simulink model "Poten"  (R2024b)
settings: Solver=FixedStepAuto  StartTime=0.0  StopTime=inf  RelTol=1e-3  EnableMultiTasking=on
libraries: stm32f4xxblockslib x2, simulink x1
settings Model: STM32="{\"AnalogInput\":[{\"ID\":\"untitled:1\"},{\"ID\":\"Poten:1\"}],\"DigitalPortRead\":[{\"ID\":\"untitled:21\"},{\"ID\":\"Poten:21\"}]}"  Creator=rew1m  LastModifiedBy=janej
settings OptimizationCC: DefaultParameterBehavior=Inlined  EnhancedBackFolding=on  PassReuseOutputArgsAs=Individual arguments  ZeroExternalMemoryAtStartup=off  ZeroInternalMemoryAtStartup=off  MaxStackSize=512  OptimizeBlockOrder=speed  DifferentSizesBufferReuse=on  OptimizationCustomize=off  EfficientTunableParamExpr=on
settings DebuggingCC: ParameterTunabilityLossMsg=error
settings HardwareCC: ProdBitPerPointer=32  ProdBitPerSizeT=32  ProdBitPerPtrDiffT=32  ProdLargestAtomicInteger=Long  ProdLargestAtomicFloat=Double  ProdWordSize=32  ProdLongLongMode=on  ProdHWDeviceType=ARM Compatible->ARM Cortex-M
settings SFSimCC: MATLABDynamicMemAlloc=off
settings RTWCC: Description=Embedded Coder  SystemTargetFile=ert.tlc  HardwareBoard=STM32G4xx Based  TemplateMakefile=ert_default_tmf  Toolchain=GNU Tools for ARM Embedded Processors
settings CodeAppCC: ForceParamTrailComments=on  IgnoreCustomStorageClasses=off  OperatorAnnotations=on  SimulinkDataObjDesc=on  SFDataObjDesc=on  InsertBlockDesc=on
settings ERTTargetCC: TargetLangStandard=C99 (ISO)  CodeReplacementLibrary=ARM Cortex-M  ExtModeTransport=3  ExtModeStaticAlloc=on  ExtModeStaticAllocSize=2048  ExtModeMexFile=ext_xcp  ExtModeIntrfLevel=Level2 - Open

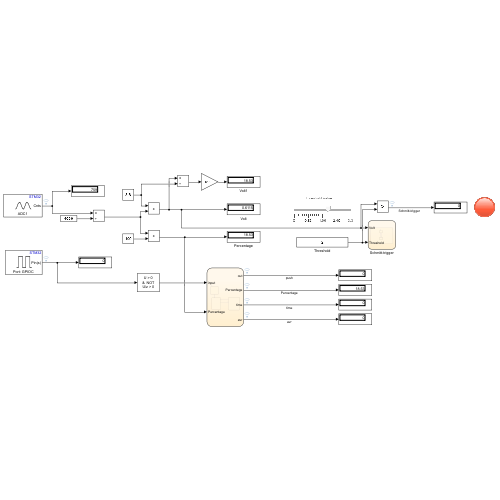
[thumbnail: Simulink's stored preview of the top-level diagram]
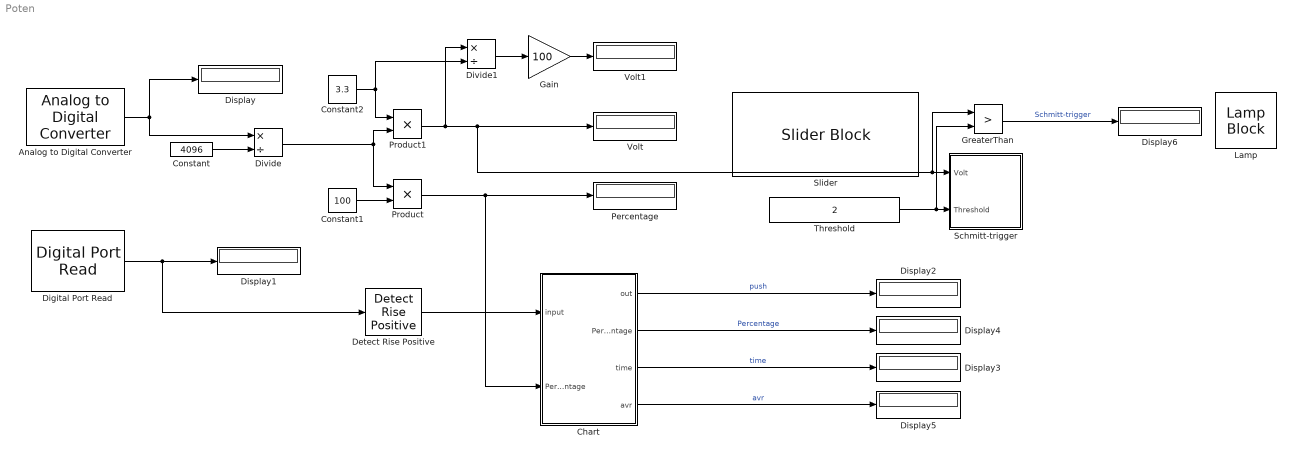
== system Poten ==
  Analog to Digital Converter : stm32f4xxblockslib/Analog to Digital Converter  ADCModule=ADC1  ConversionGroup=Regular  TriggerMode=Trigger and read  NumberOfConversions=1  EnableBufferConv=off  BufferLength=1  OutputStatus=off  SampleTime=-1  EnableSimPort=off  hoistedMaskSrc=ECSoC/ECSimCodegen/Analog to Digital Converter
  Chart : Stateflow chart  TreatAsAtomicUnit=on
  Constant : Constant  Value=4096
  Constant1 : Constant  Value=100
  Constant2 : Constant  Value=3.3
  Detect Rise Positive : simulink/Logic and Bit Operations/Detect Rise Positive  vinit=0  OutDataTypeStr=boolean
  Digital Port Read : stm32f4xxblockslib/Digital Port Read  PortName=GPIOC  PinNumber=[13]  ReadOperation=on  IOAsArray=on  SampleTime=-1  EnableSimPort=off  hoistedMaskSrc=ECSoC/ECSimCodegen/Digital Port Read
  Display{,1..6} (7 alike) : Display
  Divide : Product  Inputs=*/
  Divide1 : Product  Inputs=*/
  Gain : Gain  Gain=100
  GreaterThan : RelationalOperator  Operator=>  OutDataTypeStr=boolean  RndMeth=Simplest  InputSameDT=off
  Lamp : LampBlock  LabelPosition=Hide
  Percentage : Display
  Product : Product
  Product1 : Product
  Schmitt-trigger : Stateflow chart  TreatAsAtomicUnit=on
  Slider : SliderBlock  ScaleMax=3.3
  Threshold : Constant  Value=2
  Volt : Display
  Volt1 : Display
  wires:
  Analog to Digital Converter/1 -> Display/1, Divide/1
  Constant/1 -> Divide/2
  Divide/1 -> Product/1, Product1/2
  Constant1/1 -> Product/2
  Product/1 -> Chart/2("Percentage "), Percentage/1
  Constant2/1 -> Product1/1, Divide1/2
  Product1/1 -> GreaterThan/1, Schmitt-trigger/1(Volt), Volt/1, Divide1/1
  Divide1/1 -> Gain/1
  Gain/1 -> Volt1/1
  Digital Port Read/1 -> Detect Rise Positive/1, Display1/1
  Detect Rise Positive/1 -> Chart/1(input)
  Chart/1(out) -> Display2/1  "push"
  Chart/3(time) -> Display3/1  "time"
  GreaterThan/1 -> Display6/1  "Schmitt-trigger"
  Threshold/1 -> GreaterThan/2, Schmitt-trigger/2(Threshold)
  Chart/2(Percentage) -> Display4/1  "Percentage"
  Chart/4(avr) -> Display5/1  "avr"

== stateflow chart Poten/Schmitt-trigger ==
  state Schmitt_trigger
    state Low
      LED = 0;
    state Hight
      LED = 1;
    (default) -> Low
    Hight -> Low : [Volt < Threshold]
    Low -> Hight : [Volt > Threshold]
  (default) -> Schmitt_trigger
  data: Volt input; Threshold input; LED local

== stateflow chart Poten/Chart ==
  state Inital
    time = 0;
    out = 0;
    total = 0;
    avr = 0;
    round = 1;
  state HIGHT
    entry:
    out = 1;
    time = 0.01;
    avr = 0;
    during:
    time = time + 0.002
    Percentage = Percentage
    total = total + Percentage
    round = round + 1
  state Low
    entry:
    out = 0;
    avr = total/round
    total = 0;
    round = 0;
  (default) -> Inital
  Inital -> Low
  HIGHT -> Low : [round >= 1000]
  Low -> HIGHT : [input == 1]
  data: out output; Percentage output; input input; time output; Percentage input; avr output; total local; round local
